simulink model "test_module"  (R2023b)
settings: Solver=FixedStepAuto  StartTime=0.0  StopTime=inf  FixedStep=1  RelTol=1e-3
model workspace (MAT data in the model file):
  SL_ROS_VariableLengthArrays_MaxSizes.CommonInfo.ArrayTruncateAction = 'EmitWarning'
  SL_ROS_VariableLengthArrays_MaxSizes.MsgTypeMap = containers.Map
  SL_ROS_VariableLengthArrays_MaxSizes.MsgTypeMap.serialization.keys = {'sensor_msgs/CompressedImage', 'sensor_msgs/LaserScan'}
  SL_ROS_VariableLengthArrays_MaxSizes.MsgTypeMap.serialization.values{1}(1).PropertyName = 'data'
  SL_ROS_VariableLengthArrays_MaxSizes.MsgTypeMap.serialization.values{1}(1).DataType = 'uint8'
  SL_ROS_VariableLengthArrays_MaxSizes.MsgTypeMap.serialization.values{1}(1).MaxLength = 200000
  SL_ROS_VariableLengthArrays_MaxSizes.MsgTypeMap.serialization.values{1}(2).PropertyName = 'format'
  SL_ROS_VariableLengthArrays_MaxSizes.MsgTypeMap.serialization.values{1}(2).DataType = 'uint8'
  SL_ROS_VariableLengthArrays_MaxSizes.MsgTypeMap.serialization.values{1}(2).MaxLength = 2000
  SL_ROS_VariableLengthArrays_MaxSizes.MsgTypeMap.serialization.values{2}(1).PropertyName = 'intensities'
  SL_ROS_VariableLengthArrays_MaxSizes.MsgTypeMap.serialization.values{2}(1).DataType = 'single'
  SL_ROS_VariableLengthArrays_MaxSizes.MsgTypeMap.serialization.values{2}(1).MaxLength = 1080
  SL_ROS_VariableLengthArrays_MaxSizes.MsgTypeMap.serialization.values{2}(2).PropertyName = 'ranges'
  SL_ROS_VariableLengthArrays_MaxSizes.MsgTypeMap.serialization.values{2}(2).DataType = 'single'
  SL_ROS_VariableLengthArrays_MaxSizes.MsgTypeMap.serialization.values{2}(2).MaxLength = 1080
  SL_ROS_VariableLengthArrays_MaxSizes.MsgTypeMap.serialization.uniformity = 0
  SL_ROS_VariableLengthArrays_MaxSizes.MsgTypeMap.serialization.keyType = 'char'
  SL_ROS_VariableLengthArrays_MaxSizes.MsgTypeMap.serialization.valueType = 'any'
undefined symbols (not defined in the file or in its folder): angular, gray, linear
libraries: ros2lib x8
settings Model: Creator=bowen  LastModifiedBy=bowen
settings OptimizationCC: EnhancedBackFolding=on  PassReuseOutputArgsAs=Individual arguments  ZeroExternalMemoryAtStartup=off  ZeroInternalMemoryAtStartup=off  MaxStackSize=64  OptimizeBlockOrder=speed  DifferentSizesBufferReuse=on  OptimizationCustomize=off  EfficientTunableParamExpr=on
settings DebuggingCC: ParameterTunabilityLossMsg=error
settings SFSimCC: MATLABDynamicMemAlloc=off
settings RTWCC: Description=Embedded Coder  SystemTargetFile=ert.tlc  HardwareBoard=Robot Operating System 2 (ROS 2)  TLCOptions="-aInlineSetEventsForThisBaseRateFcn=TLC_FALSE -aSuppressMultiTaskScheduler=TLC_FALSE  -aRateBasedStepFcn=0"  TemplateMakefile=ert_default_tmf  Toolchain=Colcon Tools  TargetLang=C++
settings CodeAppCC: ForceParamTrailComments=on  IgnoreCustomStorageClasses=off  OperatorAnnotations=on  SimulinkDataObjDesc=on  SFDataObjDesc=on  InsertBlockDesc=on
settings ERTTargetCC: CodeInterfacePackaging=C++ class  RootIOFormat=Structure reference

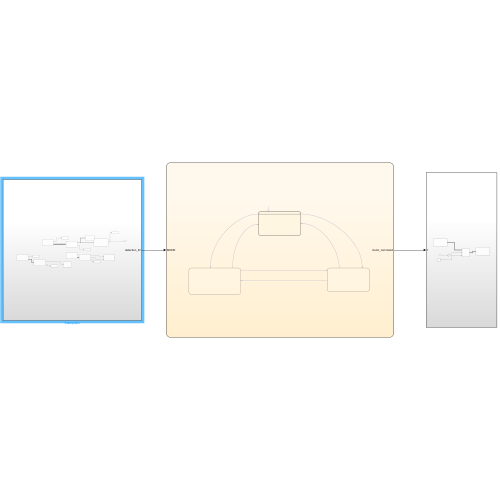
[thumbnail: Simulink's stored preview of the top-level diagram]
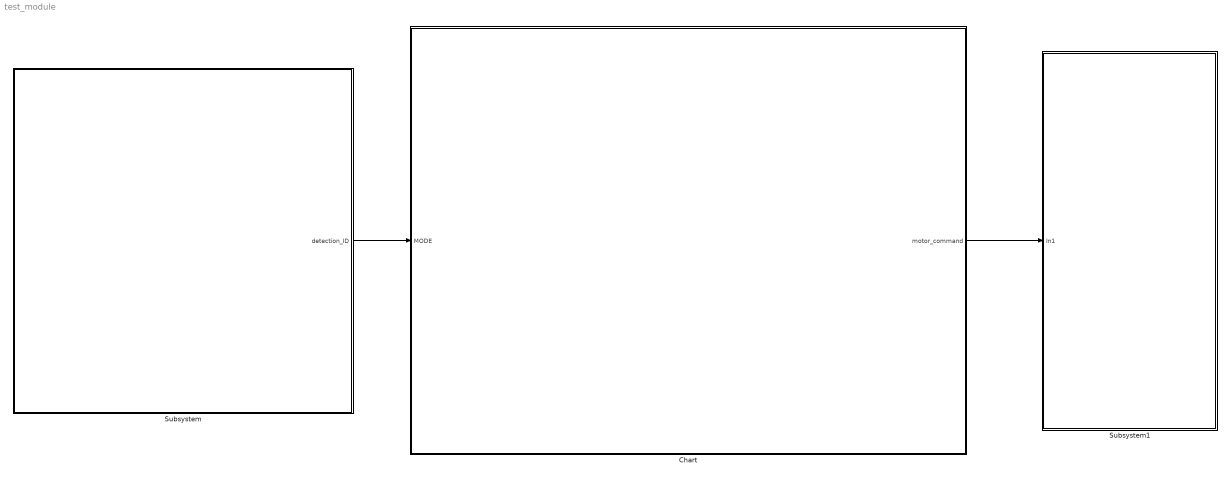
== system test_module ==
  Chart : Stateflow chart  TreatAsAtomicUnit=on
  Subsystem : Subsystem
  Subsystem1 : Subsystem
  wires:
  Subsystem/1(detection_ID) -> Chart/1(MODE)
  Chart/1(motor_command) -> Subsystem1/1(In1)

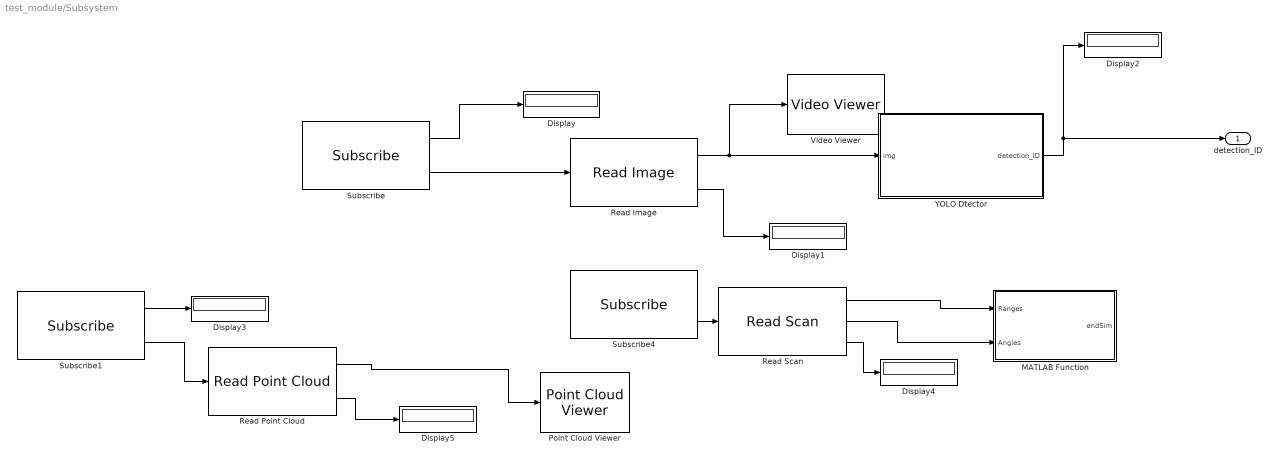
== system test_module/Subsystem ==
  Display{,1..5} (6 alike) : Display
  MATLAB Function : MATLAB Function  TreatAsAtomicUnit=on
  Point Cloud Viewer : PointCloudViewer  FigPos=[30 1000 1375 820]
  Read Image : ros2lib/Read Image  MaximumImageSize=[480, 640]  ImageEncoding=rgb8  ShowAlphaOutput=off  ShowErrorCodeOutput=on  VariableSizeOutputs=on
  Read Point Cloud : ros2lib/Read Point Cloud  MaximumPointCloudSize=[480, 640]  PreserveStructure=off  ShowRGBOutput=off  ShowIntensityOutput=off  ShowErrorCodeOutput=on  VariableSizeOutputs=off
  Read Scan : ros2lib/Read Scan  MaximumArrayLength=1080  ShowAnglesOutput=on  ShowIntensityOutput=off  ShowErrorCodeOutput=on  VariableSizeOutputs=off
  Subscribe : ros2lib/Subscribe  topicSource=Select from ROS network  topic=/depth_cam/rgb/image_raw/compressed  messageType=sensor_msgs/CompressedImage  sampleTime=-1  QOSHistory=Keep last  QOSDepth=1  QOSReliability=Best effort  QOSDurability=Volatile
  Subscribe1 : ros2lib/Subscribe  topicSource=Select from ROS network  topic=/depth_cam/depth/points  messageType=sensor_msgs/PointCloud2  sampleTime=-1  QOSHistory=Keep last  QOSDepth=1  QOSReliability=Reliable  QOSDurability=Volatile
  Subscribe4 : ros2lib/Subscribe  topicSource=Select from ROS network  topic=/scan  messageType=sensor_msgs/LaserScan  sampleTime=-1  QOSHistory=Keep last  QOSDepth=1  QOSReliability=Best effort  QOSDurability=Volatile
  Video Viewer : VideoViewer  colormapValue=gray(256)  FigPos=[962 1029 958 920]
  YOLO Dtector : MATLAB Function  TreatAsAtomicUnit=on
  detection_ID : Outport
  wires:
  YOLO Dtector/1(detection_ID) -> Display2/1, detection_ID/1
  Read Image/2 -> Display1/1
  Read Image/1 -> YOLO Dtector/1(img), Video Viewer/1
  Subscribe/2 -> Read Image/1
  Subscribe/1 -> Display/1
  Read Scan/3 -> Display4/1
  Read Scan/1 -> MATLAB Function/1(Ranges)
  Read Scan/2 -> MATLAB Function/2(Angles)
  Subscribe1/1 -> Display3/1
  Subscribe1/2 -> Read Point Cloud/1
  Read Point Cloud/1 -> Point Cloud Viewer/1
  Read Point Cloud/2 -> Display5/1
  Subscribe4/2 -> Read Scan/1

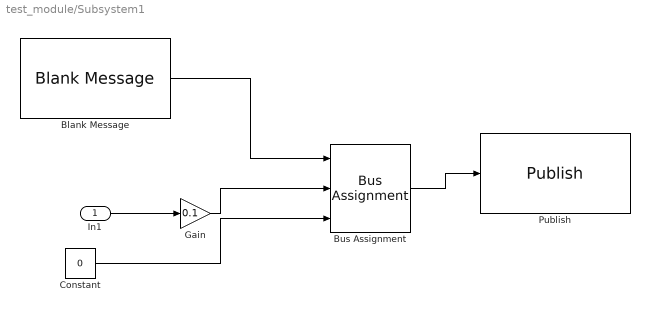
== system test_module/Subsystem1 ==
  In1 : Inport
  Blank Message : ros2lib/Blank Message  messageClass=Message  entityType=geometry_msgs/Twist  messageType=geometry_msgs/Twist  SampleTime=1
  Bus Assignment : BusAssignment  AssignedSignals=linear.x,angular.z
  Constant : Constant  Value=0
  Gain : Gain  Gain=0.1
  Publish : ros2lib/Publish  topicSource=Select from ROS network  topic=/controller/cmd_vel  messageType=geometry_msgs/Twist  QOSHistory=Keep last  QOSDepth=1  QOSReliability=Reliable  QOSDurability=Volatile
  wires:
  Blank Message/1 -> Bus Assignment/1
  In1/1 -> Gain/1
  Constant/1 -> Bus Assignment/3
  Bus Assignment/1 -> Publish/1
  Gain/1 -> Bus Assignment/2

== matlab function test_module/Subsystem/MATLAB Function ==
  data: Ranges input; Angles input; endSim output
function endSim = plotXY(Ranges, Angles)
% Read Scan block will output all zeros until the Subscriber blocks 
% outputs a message  
endSim = any(Ranges>0);
if endSim
    x = Ranges.*cos(Angles);
    y = Ranges.*sin(Angles);
    % only return finite values
    xValid = x(isfinite(x));
    yValid = y(isfinite(y));

    plot(0, 0, 'r.', 'MarkerSize', 25);
    plot(xValid,yValid,marker=".",LineStyle="none", MarkerSize=8)
    
    title('Laser Scan')
    xlabel("X")
    ylabel("Y")
    set(gca, 'YDir','reverse')
    grid on
    axis equal
    ylim([-3 3])
    xlim([-3 3])
    view([90 -90])
end

== matlab function test_module/Subsystem/YOLO Dtector ==
  data: img input; detection_ID output
function detection_ID = detect_yolov8(img)
% This block's only job is to call the external wrapper script.

% Declare that our external .m file should be run by the MATLAB engine.
coder.extrinsic('yolo_detection_wrapper');

% Always pre-initialize outputs to define their type and size for Simulink.
detection_ID = 0;

% Call the wrapper function to do all the hard work.
% It takes the image and returns a simple number (0, 1, or 2).
detection_ID = yolo_detection_wrapper(img);

end

== stateflow chart test_module/Chart ==
  state Idle
    entry:
    motor_command = 0
  state Move_Forward
    entry:
    motor_command = 1
  state Move_Backward
    entry:
    motor_command = -1
  (default) -> Idle
  Idle -> Move_Forward [order 1] : [MODE==1]
  Idle -> Move_Backward [order 2] : [MODE==2]
  Move_Backward -> Idle [order 1] : after(3, sec)[MODE == 0]
  Move_Forward -> Idle [order 1] : after(3, sec)[MODE == 0]
  Move_Forward -> Move_Backward [order 2] : after(3,sec)[MODE==2]
  Move_Backward -> Move_Forward [order 2] : after(3, sec)[MODE==1]
  data: MODE input; motor_command output
